simulink model "MSM_strain_wave_actuator"  (R2024b)
settings: Solver=ode23t  StartTime=0.0  StopTime=SIMULATION_TIME  FixedStep=MAX_TIME_STEP  MaxStep=MAX_TIME_STEP  RelTol=1e-3  AbsTol=1e-3  EnableMultiTasking=on
PreLoadFcn:
  | linear_mechanism = Simulink.Variant('motion_type == "linear"');
  | rotary_mechanism = Simulink.Variant('motion_type == "rotary"');
values from neighbouring files (symbols this model uses):
  action = round(out.position_data.Data(:,5))    [msm_tooth_training_run.m]
  contact_ratio = tooth_plates_cnt / (2 * (t_a / t_b + 1))    (= 2)    [MSM_mechanism_simulation_properties.m]
  contraction_initial = -msm_length * e_initial    (= -0.001)    [MSM_mechanism_simulation_properties.m]
  controller_type_vec = zeros(tooth_plates_cnt, 1)    [MSM_mechanism_simulation_properties.m]
  controller_velocity_setpoint = velocity_iter    [controller_mass_comparison_runs.m]
  disk_diameter = disk_teeth_count * tooth_pitch / pi    [MSM_mechanism_simulation_properties.m]    (also in msm_sim_runs_for_pid.m = evalin('base','disk_diameter'); save_sim_result.m = evalin('base','disk_diameter'))
  disk_height = 2.5e-4    (= 0.00025)    [MSM_mechanism_simulation_properties.m]    (also in get_tooth_properties.m)
  feedback_threshold = 1.025    [MSM_mechanism_simulation_properties.m]    (also in get_tooth_properties.m; msm_sim_runs_for_pid.m = evalin('base','feedback_threshold'))
  force_control_coeff = 1.0    (= 1)    [MSM_mechanism_simulation_properties.m]
  HALT_VELOCITY = 0.2    [MSM_mechanism_simulation_properties.m]    (also in get_tooth_properties.m)
  in_pair_angle_tooth_plates_pitch = 2*pi * (-2*tooth_pitch + in_pair_tooth_plates_pitch) / (pi*disk_diameter)    (= 0.412285714286)    [MSM_mechanism_simulation_properties.m]    (also in get_tooth_properties.m = 2*pi * (-2*tooth_pitch + in_pair_tooth_plates_pitch) / (pi*t)
  MAX_OVERLOAD_VELOCITY = 100    [MSM_mechanism_simulation_properties.m]    (also in get_tooth_properties.m)
  MAX_POSITION = rack_initial_position + max_teeth_passed * tooth_plates_cnt * angle_single_tooth_step    [MSM_mechanism_simulation_properties.m]    (also in get_tooth_properties.m)
  MAX_TIME_STEP = 5e-6    (= 5e-06)    [MSM_mechanism_simulation_properties.m]
  min_tooth_motion_range = -msm_length * allowed_elongation    (= -0.001)    [MSM_mechanism_simulation_properties.m]
  motion_type_number = NaN    [MSM_mechanism_simulation_properties.m]
  next_vec_fraction = -0.05    [MSM_mechanism_simulation_properties.m]    (also in msm_sim_runs_for_pid.m = evalin('base','next_vec_fraction'))
  obs_matrix = zeros(tooth_plates_cnt, obs_matrix_size)    [MSM_mechanism_simulation_properties.m]
  one_side_absolute_offset = one_side_elongation_capacity * msm_length    (= 0.0001)    [MSM_mechanism_simulation_properties.m]
  rack_coulumb_friction = 0.05    [MSM_mechanism_simulation_properties.m]
  rack_initial_position = rack_initial_position + 4*angle_single_tooth_step    (= 0.0554357142857)    [MSM_mechanism_simulation_properties.m]    (also in get_tooth_properties.m = rack_initial_position + 4*angle_single_tooth_step)
  rack_mass = 4e-3    (= 0.004)    [MSM_mechanism_simulation_properties.m]
  rotational_rack_coulumb_friction = rack_coulumb_friction * disk_diameter    (= 0.00175)    [MSM_mechanism_simulation_properties.m]
  SIMULATION_TIME = 0.06    [MSM_mechanism_simulation_properties.m]    (also in msm_actuation_time_sensetivity.m = 0.04; msm_sim_runs_for_pid.m = evalin('base','SIMULATION_TIME'); msm_simulation_run.m = 0.08; msm_tooth_training_run.m = 0.04)
  swing_block_tooth_plates_pitch = 2 * tooth_pitch * 22 + tooth_pitch / tooth_plates_cnt    (= 0.0172575)    [MSM_mechanism_simulation_properties.m]    (also in get_tooth_properties.m = 2 * tooth_pitch * 22 + tooth_pitch / tooth_plates_cnt)
  tooth_disk_mass = 5e-3    (= 0.005)    [MSM_mechanism_simulation_properties.m]
  tooth_pitch = tooth_pitch * tooth_size_modifier    (= 0.00039)    [MSM_mechanism_simulation_properties.m]    (also in get_tooth_properties.m = 0.00024661; msm_sim_runs_for_pid.m = evalin('base','tooth_pitch'); save_sim_result.m = evalin('base','tooth_pitch'))
  tooth_plates_cnt = 4    [MSM_mechanism_simulation_properties.m]    (also in MSM_simulation_data_processing.m = sim_data.tooth_plates_cnt; msm_actuation_time_sensetivity.m = plates_cnt_iter; msm_sim_runs_for_pid.m = evalin('base','tooth_plates_cnt'); msm_simulation_run.m = plates_cnt_iter)
  tooth_plates_pitch = tooth_pitch * 12 + tooth_pitch / tooth_plates_cnt    (= 0.0047775)    [MSM_mechanism_simulation_properties.m]    (also in get_tooth_properties.m = tooth_pitch * 12 + tooth_pitch / tooth_plates_cnt)
  useful_load = -2    [MSM_mechanism_simulation_properties.m]    (also in controller_mass_comparison_runs.m)
  useful_mass = 0.0001    [MSM_mechanism_simulation_properties.m]    (also in controller_mass_comparison_runs.m = 0.025)
  VALIDATION_START_TIME = 0.25*SIMULATION_TIME    (= 0.015)    [MSM_mechanism_simulation_properties.m]
  Z = griddata(x,y,z,X,Y)    [MSM_simulation_data_processing.m]
undefined symbols (not defined in the file or in its folder): controller_amplitude_setpoint, controller_desired_profile_type, controller_frequency_setpoint, controller_loop_type, enable_neighbours_obs, enable_vel_setpoint, external_control_value, has_external_controller, initial_spike_force, random_delay_probablity, random_switch_probability, sim_state_code, simulation_pause_time, X, Y
libraries: sm_lib x141, MSM_element x72, Flat_tooth_plate x36, Rotary_tooth_plate x36, Swing_mechanism x18, nesl_utility x16, simulink x10, fl_lib x9, rllib x7, spsMeanLib x2, slctrl_autotuning x2, slpidlib x1
(part 7 of 7)

== matlab function MSM_strain_wave_actuator/controller/Closed//open loop simple feedback controller1/MATLAB Function ==
  data: time input; output_vector output; loop_type input; cycle_length input; initial_idle_time input; feedback_threshold input; next_vec_fraction input; feedback input; rack_position input; ticks_cnt input; currently_active input; tooth_plates_cnt parameter; cur_active_output output; tooth_pitch parameter; rack_initial_position parameter; disk_diameter parameter; motion_type_number parameter; contact_ratio parameter
function [output_vector, cur_active_output]   = fcn(time, loop_type, cycle_length, ... % open loop inputs
    initial_idle_time, ... % input for stable simulation data
    feedback_threshold, next_vec_fraction,...
    feedback, rack_position,  ticks_cnt, currently_active,... % closed loop inputs (two different feedback methods)
    tooth_plates_cnt,  tooth_pitch, rack_initial_position, disk_diameter, motion_type_number, contact_ratio) % egagement and disengagement timings  % this line contains parameters

% loop_type - lower than 0.5 is open loop, any value higher than 0.5 is a closed loop
% open loop parameters:
% cycle_length - duration of the actuation cycle of the whole plate set
% closed loop parameters:
% feedback, position feedback in range [0, 1], where 0 is fully contracted and 1 is fully extended
% motion_type_number: 0 == linear, 1 == rotary.
% next_vec_fraction - defines the disengagement timing for the last tooth,
% Positive value leads to earlier disengagement and negative value to the later disengagement

output_vector = zeros(tooth_plates_cnt, 1);
cur_active_output = currently_active;
tick = 0;

if time < initial_idle_time; return; end

if loop_type < 0.5 % open loop
    frac = mod(abs(time / cycle_length), 1);
    cur_active = -1;
    for i = 1:tooth_plates_cnt
        if frac < i / tooth_plates_cnt
            output_vector(i) = 1;
            if currently_active ~= i; tick = 1; end
            cur_active = i;
            cur_active_output = i;
            break;
        end
    end
    %if ticks_cnt > 0.5
    output_vector(cur_active_output) = 1; % this line added without testing. TODO test if it works properly
    output_vector(get_following_active_vec(cur_active, tooth_plates_cnt)) = 1; % TODO: modify open loop to support contact ratio
    %end
    return;
end

% ===== closed loop section =====

% next_active_vec = get_following_active_vec(currently_active, tooth_plates_cnt);

% --- Feedbacks based on complition of extension of a previous MSM element
% (so the next element is considered as "active"

% - original switch:
% if feedback(currently_active) > feedback_threshold %% 0.9 for the big pitch, over 0.9 for the small pitch
%     cur_active_output = next_active_vec(1);
%     tick = 1;
% end

% - modified switch: --- has problems at low loads where several active
% elements start to compete with each other
% for i = 1 : tooth_plates_cnt
%     if feedback(i) > feedback_threshold %% 0.9 for the big pitch, over 0.9 for the small pitch
%         tmp_next_active = get_following_active_vec(i, tooth_plates_cnt);
%         cur_active_output = tmp_next_active(1);
%         next_active_vec = get_following_active_vec(tmp_next_active(1), tooth_plates_cnt);
%         tick = 1;
%     end
% end


% --- rack feedback ---  Active element is determined based on the rack/disk position

% next_vec_fraction = 0; % before next_vec_fraction was a parameter, it had been defined on this line
for i = 2 : tooth_plates_cnt + 1
    if motion_type_number == 0 % linear case
        cur_cycle = rem(abs(rack_position - rack_initial_position - tooth_pitch), tooth_pitch); % getting reminder of the division. the substraction of the extra tooth_pitch is needed to guarantee first element push at the initial state
        switch_threshold = (i - 1) * tooth_pitch / tooth_plates_cnt - (1 - feedback_threshold) * tooth_pitch / tooth_plates_cnt; % the second term is to eliminate dead points
    else % rotary case % fi_max = 2*tooth_pitch / disk_diameter;  % - 2*tooth_pitch / disk_diameter
        cur_cycle = rem(abs(rack_position - rack_initial_position + 2*tooth_pitch / disk_diameter), 2*tooth_pitch / disk_diameter); % the extra addition of 2*tooth_pitch / disk_diamete has the same logic as for linear case (see the comments above)
        switch_threshold = (i - 1) * 2 * tooth_pitch / tooth_plates_cnt / disk_diameter - (1 - feedback_threshold) * 2 * tooth_pitch / tooth_plates_cnt / disk_diameter;
    end
    if cur_cycle < switch_threshold || i == tooth_plates_cnt + 1 % the second condition is a new part
        if i == tooth_plates_cnt + 1
            i = 1;
        end
        currently_active = i;
        cur_active_output = i; % questionable
        break
    end
end

next_active_vec = get_following_active_vec(currently_active, tooth_plates_cnt, contact_ratio, next_vec_fraction); % CR is concidered
% next_active_vec = get_following_active_vec(currently_active, tooth_plates_cnt); % this call always engages 50% of the teeth

% if ticks_cnt > 0.5
output_vector(next_active_vec) = 1;
% end
output_vector(cur_active_output) = 1;
% if ticks_cnt > 0.5
%     cur_active_output = next_active_vec(1);
% end

end

function following_active_vec = get_following_active_vec(cur_active, plates_cnt, contact_ratio, fraction)
% fraction - optional; is in [0; 1] range
% contact_ratio - optional; if contact ratio is unknown, the N/2 value can be used with 0 fraction.
% The performance will be higher if the contact ration is given. (N = tooth_plates_cnt)
    if nargin < 3
        iteration_range = cur_active + 1 : cur_active + round(plates_cnt / 2) - 1; % cur_active + ceil(plates_cnt / 2) - 1
    else
        fraction_tooth = ceil(mod(contact_ratio, 1) - fraction - 1e-6);
        % if fraction_tooth < 0; fraction_tooth = 0; end  % in case fraction ratio is too big. this line has been never tested
        iteration_range = cur_active + 1 : cur_active + round(floor(contact_ratio)) - 1 + fraction_tooth;
    end
    following_active_vec = 1:0; % creating empty double vector with this line, otherwise matlab will show a data cast warning later 
    for i = 1:length(iteration_range) % otherwise the Matlab coder does not work
        new_active_val = mod(iteration_range(i), plates_cnt+1);
        if new_active_val < cur_active
            new_active_val = new_active_val + 1;
        end
        following_active_vec = [following_active_vec new_active_val];
    end
end

== matlab function MSM_strain_wave_actuator/controller/MATLAB Function ==
  data: spike input; pid_value input; delayed_pid_value input; tahn_acc input; new_pid_value output; cur_time input; mem_time input; mem_pid_value input; mem_time output; mem_pid_value output; mem_control_state input; mem_control_state output
function [new_pid_value, mem_time, mem_pid_value, mem_control_state] = fcn(spike, pid_value, delayed_pid_value, tahn_acc, cur_time, mem_time, mem_pid_value, mem_control_state)

INITIAL_DELAY = 0.004;
TIME_DELAY = 0.0008;  % delay for which the pid value is being hold
COMPENSATION_COEFF = 1.03; % 1.03 is correct for optimal pitch, 2 N load
ACC_LIMIT = 0.004; % worked with 0.002; works better with 0.004

if cur_time < INITIAL_DELAY 
    new_pid_value = pid_value;
    mem_pid_value = pid_value;
    return;
end

if spike > 0.5
    mem_time = cur_time;
    mem_control_state = 1;
    new_pid_value = delayed_pid_value * COMPENSATION_COEFF;
    return;
end

if (cur_time > mem_time + TIME_DELAY) && ( abs(tahn_acc ) > ACC_LIMIT || mem_control_state < 0.5) 
    mem_control_state = 0;
    new_pid_value = pid_value;
    return;
end

new_pid_value = pid_value * COMPENSATION_COEFF;
return;


% case (which is remaining) of: cur_time < mem_time + TIME_DELAY
%new_pid_value = mem_pid_value;



%% old working logic (with timer) actually it works BETTER that the acceleration based one, but requires precise timing guess, which might not be possible with an unknown external load
return; % to cooment out the old part

TIME_DELAY = 0.00125;  % delay for which the pid value is being hold
COMPENSATION_COEFF = 1.03; % 1.03 is correct for optimal pitch, 2 N load
if cur_time > mem_time + TIME_DELAY && spike == 0
    new_pid_value = pid_value;
    return;
end

if spike == 1
    mem_time = cur_time;
    %mem_pid_value = delayed_pid_value * COMPENSATION_COEFF;
    %new_pid_value = mem_pid_value;
    new_pid_value = delayed_pid_value * COMPENSATION_COEFF;
    return;
end

% case (which is remaining) of: cur_time < mem_time + TIME_DELAY
%new_pid_value = mem_pid_value;
new_pid_value = pid_value * COMPENSATION_COEFF;

== matlab function MSM_strain_wave_actuator/controller/Blocking PID value ==
  data: pid_input input; forward_pid output; reverse_pid output; no_blocking input
function [forward_pid, reverse_pid] = fcn(pid_input, no_blocking)
% function outputs a small control signal for all non-pushing teeth for
% breaking if the pid_input value is too small

% params:
% pid_input : float
% no_blocking : bool (0/1), if true prhobits blocking counteraction

% previously somehow worked with these values:
%PID_VALUE_LIMIT = 1.0; % function starts to output non-zero value if pid_input is within this range
%MAX_BLOCKING_OUTPUT_VALUE = 1.0; % worked well with 1.0 value


PID_VALUE_LIMIT = 0.4; % function starts to output non-zero value if pid_input is within this range
MAX_BLOCKING_OUTPUT_VALUE = 0.5; % worked well with 1.0 value

if pid_input > PID_VALUE_LIMIT
    reverse_pid = 0;
elseif pid_input < 0
    reverse_pid = -pid_input; % + MAX_BLOCKING_OUTPUT_VALUE;
else    
    if no_blocking > 0.5
        reverse_pid = 0;
    else
        reverse_pid = (PID_VALUE_LIMIT - abs(pid_input)) * MAX_BLOCKING_OUTPUT_VALUE / PID_VALUE_LIMIT; % mapping output value to the desired range, linear dependency
    end
end

pid_input = -pid_input;

if pid_input > PID_VALUE_LIMIT
    forward_pid = 0;
elseif pid_input < 0
    forward_pid = -pid_input; % + MAX_BLOCKING_OUTPUT_VALUE;
else  
    if no_blocking > 0.5
        forward_pid = 0;
    else
        forward_pid = (PID_VALUE_LIMIT - abs(pid_input)) * MAX_BLOCKING_OUTPUT_VALUE / PID_VALUE_LIMIT; % mapping output value to the desired range, linear dependency
    end
end


end

== matlab function MSM_strain_wave_actuator/controller/reward function1 ==
  data: stop_sim_code input; rack_abs_pos input; instant_rack_vel input; controller_velocity_setpoint input; reward output; isdone output; tooth_plates_cnt parameter; sim_state_code parameter; rack_initial_position parameter; enable_vel_setpoint parameter
function [reward,isdone] = reward(stop_sim_code, rack_abs_pos, instant_rack_vel,  controller_velocity_setpoint,...
    tooth_plates_cnt, sim_state_code, rack_initial_position, enable_vel_setpoint) % params

%instant_rack_vel = observation(3 * tooth_plates_cnt + 2);

% if time < 1e-7
%     rack_vel = instant_rack_vel;
% else
%     rack_vel = -rack_abs_pos / time; % measuring rack average velocity; Negative value taken
% end

% calculate reward value
reward = 0;

% penalty for staying still:
% if abs(instant_rack_vel) < 0.001
%     reward = reward - 1;
% end
% if instant_rack_vel > -0.001
%     reward = reward - 0.2;
% end

% if sum(action > 0.5) > 0.75 * tooth_plates_cnt
%     reward = reward - 10; % punish for too many active MSM elements at a time
% end
if enable_vel_setpoint % the reward is computed differently in case a velocity setpoint is followed
    reward = -(abs(instant_rack_vel - controller_velocity_setpoint)); % in ideal case reward is zero
end


% done if either failed (crashed) or succeeded
isdone = boolean(stop_sim_code);

== matlab function MSM_strain_wave_actuator/Count frequency ==
  data: time input; actuator_frequency output; ticks input; single_element_frequency output; tooth_plates_cnt parameter
function [actuator_frequency, single_element_frequency] = fcn(time, ticks, tooth_plates_cnt)

if time == 0 || ticks == 0
    actuator_frequency = 0;
    single_element_frequency = 0;
    return;
end

actuator_frequency = ticks / time;
single_element_frequency = actuator_frequency / tooth_plates_cnt;

== matlab function MSM_strain_wave_actuator/Subsystem/Single element frequency ==
  data: cur_rack_position input; frequency output; time input; rack_initial_position parameter; tooth_pitch parameter
function frequency = fcn(cur_rack_position, time, rack_initial_position, tooth_pitch)
% frequncy in Hz


if time < 1e-3
    frequency = 0;
    return;
end

frequency = abs(cur_rack_position - rack_initial_position) / time / tooth_pitch;

== matlab function MSM_strain_wave_actuator/controller/Closed//open loop simple feedback controller DIRECTION SWITCH IS BLOCKED!!!!/MATLAB Function ==
  data: time input; output_vector output; loop_type input; cycle_length input; initial_idle_time input; feedback_threshold input; next_vec_fraction input; feedback input; rack_position input; velocity_direction input; ticks_cnt input; currently_active input; tooth_plates_cnt parameter; cur_active_output output; tooth_pitch parameter; rack_initial_position parameter; disk_diameter parameter; motion_type_number parameter; contact_ratio parameter
function [output_vector, cur_active_output]   = fcn(time, loop_type, cycle_length, ... % open loop inputs
    initial_idle_time, ... % input for stable simulation data
    feedback_threshold, next_vec_fraction,...
    feedback, rack_position, velocity_direction, ticks_cnt, currently_active,... % closed loop inputs (two different feedback methods)
    tooth_plates_cnt,  tooth_pitch, rack_initial_position, disk_diameter, motion_type_number, contact_ratio) % egagement and disengagement timings  % this line contains parameters

% loop_type - lower than 0.5 is open loop, any value higher than 0.5 is a closed loop
% open loop parameters:
% cycle_length - duration of the actuation cycle of the whole plate set
% closed loop parameters:
% feedback, position feedback in range [0, 1], where 0 is fully contracted and 1 is fully extended
% motion_type_number: 0 == linear, 1 == rotary.
% next_vec_fraction - defines the disengagement timing for the last tooth,
% Positive value leads to earlier disengagement and negative value to the later disengagement

output_vector = zeros(tooth_plates_cnt, 1);
cur_active_output = currently_active;
tick = 0;

if time < initial_idle_time; return; end

if loop_type < 0.5 % open loop === NOTE: OPEN LOOP MIGHT NOT WORK CORRECTLY WHEN THE VELOCITY SETPOINT IS POSITIVE === TODO: fix this issue
    frac = mod(abs(time / cycle_length), 1);
    cur_active = -1;
    for i = 1:tooth_plates_cnt
        if frac < i / tooth_plates_cnt
            output_vector(i) = 1;
            if currently_active ~= i; tick = 1; end
            cur_active = i;
            cur_active_output = i;
            break;
        end
    end

    output_vector(cur_active_output) = 1; % this line added without testing. TODO test if it works properly

    % the following line enables the second tooth to be actuated
    % output_vector(get_following_active_vec(cur_active, tooth_plates_cnt, velocity_direction)) = 1; % TODO: modify open loop to support contact ratio

    return;
end

% ===== closed loop section =====

% next_active_vec = get_following_active_vec(currently_active, tooth_plates_cnt);

% --- Feedbacks based on complition of extension of a previous MSM element
% (so the next element is considered as "active"

% - original switch:
% if feedback(currently_active) > feedback_threshold %% 0.9 for the big pitch, over 0.9 for the small pitch
%     cur_active_output = next_active_vec(1);
%     tick = 1;
% end

% - modified switch: --- has problems at low loads where several active
% elements start to compete with each other
% for i = 1 : tooth_plates_cnt
%     if feedback(i) > feedback_threshold %% 0.9 for the big pitch, over 0.9 for the small pitch
%         tmp_next_active = get_following_active_vec(i, tooth_plates_cnt);
%         cur_active_output = tmp_next_active(1);
%         next_active_vec = get_following_active_vec(tmp_next_active(1), tooth_plates_cnt);
%         tick = 1;
%     end
% end


% --- rack feedback ---  Active element is determined based on the rack/disk position

% next_vec_fraction = 0; % before next_vec_fraction was a parameter, it had been defined on this line
% NOTE: this algorithm is reworked and simplified in python version
for i = 2 : tooth_plates_cnt + 1
    cur_offset = rack_position - rack_initial_position;
    quotinent = fix(cur_offset/tooth_pitch);
    if motion_type_number == 0 % linear case
        % cur_cycle = rem(abs(rack_position - rack_initial_position - tooth_pitch), tooth_pitch); % getting reminder of the division. the substraction of the extra tooth_pitch is needed to guarantee first element push at the initial state
        cur_cycle = rem(abs(cur_offset - (quotinent + 2)*tooth_pitch), tooth_pitch); % getting remainder of the division. the substraction of the extra tooth_pitch is needed to guarantee first element push at the initial state
        switch_threshold = (i - 1) * tooth_pitch / tooth_plates_cnt - (1 - feedback_threshold) * tooth_pitch / tooth_plates_cnt; % the second term is to eliminate dead points
    else % rotary case % fi_max = 2*tooth_pitch / disk_diameter;  % - 2*tooth_pitch / disk_diameter
        cur_cycle = rem(abs(cur_offset + 2*tooth_pitch / disk_diameter), 2*tooth_pitch / disk_diameter); % the extra addition of 2*tooth_pitch / disk_diamete has the same logic as for linear case (see the comments above)
        switch_threshold = (i - 1) * 2 * tooth_pitch / tooth_plates_cnt / disk_diameter - (1 - feedback_threshold) * 2 * tooth_pitch / tooth_plates_cnt / disk_diameter;
    end
    if cur_cycle < switch_threshold || i == tooth_plates_cnt + 1 % the second condition is a new part
        if i == tooth_plates_cnt + 1
            i = 1;
        end
        currently_active = i;
        cur_active_output = i; % questionable
        break
    end
end
% velocity_direction

% motion in the opposite direction  --- TODO ---
hardcode_conversion_vec = [3 4 1 2]; % conversts direct motion index into the inverse motion index
if velocity_direction > 0 && false % NOTE!!! SWITCH OF DIRECTION IS BLOCKED CURRENTLY
    currently_active = hardcode_conversion_vec(currently_active); % TODO: a generalized case should be implemented
    cur_active_output = hardcode_conversion_vec(cur_active_output);
end

next_active_vec = get_following_active_vec(currently_active, tooth_plates_cnt, velocity_direction, contact_ratio, next_vec_fraction); % CR is concidered
% next_active_vec = get_following_active_vec(currently_active, tooth_plates_cnt); % this call always engages 50% of the teeth

output_vector(next_active_vec) = 1;
output_vector(cur_active_output) = 1;

end

function following_active_vec = get_following_active_vec(cur_active, plates_cnt, velocity_direction, contact_ratio, fraction)
% fraction - optional; is in [0; 1] range
% contact_ratio - optional; if contact ratio is unknown, the N/2 value can be used with 0 fraction.
% The performance will be higher if the contact ration is given. (N = tooth_plates_cnt)
    if nargin < 4 % --- TODO this case has not been tested and probably does not work ---
        iteration_range = (cur_active + 1) : (cur_active + round(plates_cnt / 2) - 1); % cur_active + ceil(plates_cnt / 2) - 1
        % if velocity_direction > 0 % in case of inverse direction 
        %     iteration_range = (cur_active - 1) : (cur_active - round(plates_cnt / 2) + 1);
        % end
    else
        fraction_tooth = ceil(mod(contact_ratio, 1) - fraction - 1e-6);
        % if fraction_tooth < 0; fraction_tooth = 0; end  % in case fraction ratio is too big. this line has been never tested
        %if velocity_direction < 0 % in case of forward direction
            iteration_range = (cur_active + 1) : (cur_active + round(floor(contact_ratio)) - 1 + fraction_tooth);
        %else % in case of inverse direction
            %iteration_range = (cur_active - round(floor(contact_ratio)) + 1 - fraction_tooth) : (cur_active - 1);
        %end
    end
    % --- following works well for both direct and inverse direction --- 
    % no idea why it does work, just magic
    following_active_vec = 1:0; % creating empty double vector with this line, otherwise matlab will show a data cast warning later 
    for i = 1:length(iteration_range) % otherwise the Matlab coder does not work
        new_active_val = mod(iteration_range(i), plates_cnt+1);
        if new_active_val < cur_active
            new_active_val = new_active_val + 1;
        end
        following_active_vec = [following_active_vec new_active_val];
    end
end

%% --- original function, potentially has an error with 1 : cur_active
% function following_active_vec = get_following_active_vec(cur_active, plates_cnt, contact_ratio, fraction)
% % fraction - optional; is in [0; 1] range
% % contact_ratio - optional; if contact ratio is unknown, the N/2 value can be used with 0 fraction.
% % The performance will be higher if the contact ration is given. (N = tooth_plates_cnt)
%     if nargin < 3
%         iteration_range = cur_active + 1 : cur_active + round(plates_cnt / 2) - 1; % cur_active + ceil(plates_cnt / 2) - 1
%     else
%         fraction_tooth = ceil(mod(contact_ratio, 1) - fraction - 1e-6);
%         % if fraction_tooth < 0; fraction_tooth = 0; end  % in case fraction ratio is too big. this line has been never tested
%         iteration_range = cur_active + 1 : cur_active + round(floor(contact_ratio)) - 1 + fraction_tooth;
%     end
%     following_active_vec = 1:0; % creating empty double vector with this line, otherwise matlab will show a data cast warning later 
%     for i = 1:length(iteration_range) % otherwise the Matlab coder does not work
%         new_active_val = mod(iteration_range(i), plates_cnt+1);
%         if new_active_val < cur_active
%             new_active_val = new_active_val + 1;
%         end
%         following_active_vec = [following_active_vec new_active_val];
%     end
% end

== matlab function MSM_strain_wave_actuator/ /max of vector ==
  data: u input; y output
function y = fcn(u)

y = max(u);

== matlab function MSM_strain_wave_actuator/Rack type variant subsystem/Linear_rack/Single element frequency ==
  data: cur_rack_position input; frequency output; time input; rack_initial_position parameter; tooth_pitch parameter
function frequency = fcn(cur_rack_position, time, rack_initial_position, tooth_pitch)
% frequncy in Hz


if time < 1e-3
    frequency = 0;
    return;
end

frequency = abs(cur_rack_position - rack_initial_position) / time / tooth_pitch;
